simulink model "SMO_HFI_FOC"  (R2025b)
settings: Solver=FixedStepDiscrete  StartTime=0.0  StopTime=0.5  FixedStep=2e-05  RelTol=1e-3
settings Model: Creator=14420  LastModifiedBy=14420
settings DataIOCC: SaveOutput=off  SaveTime=off
settings DebuggingCC: AlgebraicLoopMsg=error

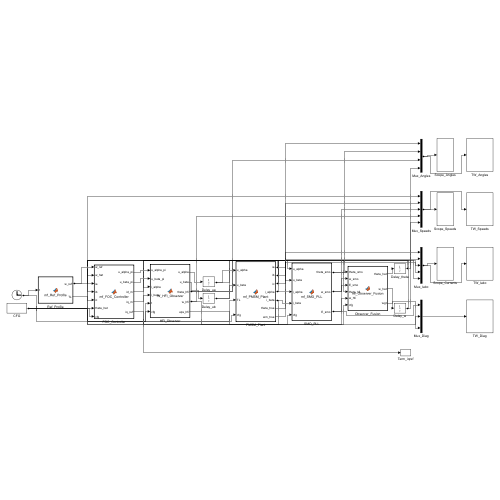
[thumbnail: Simulink's stored preview of the top-level diagram]
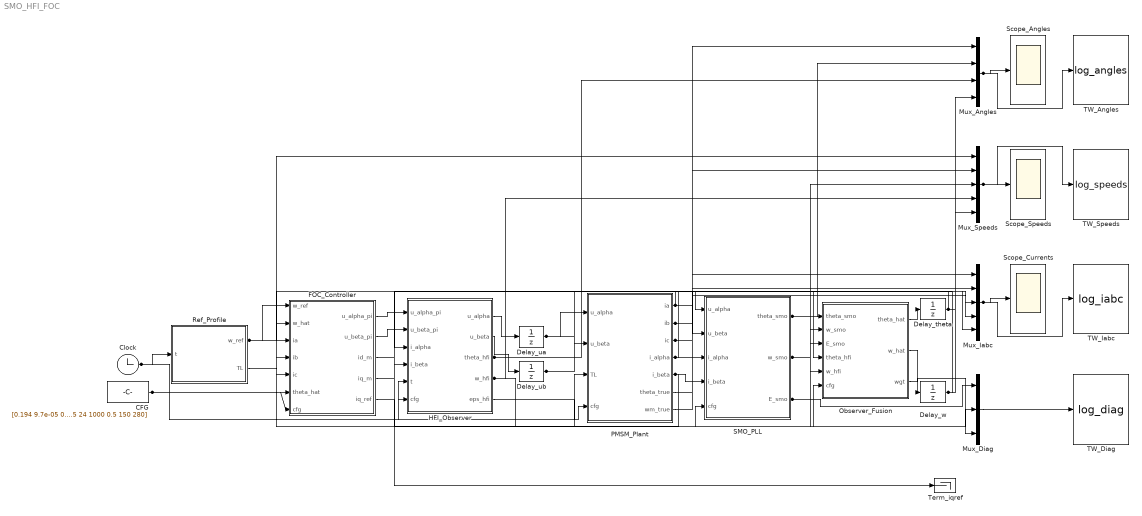
== system SMO_HFI_FOC ==
  CFG : Constant  Value=[0.194 9.7e-05 0.000145 0.015152 4 0.0006214 0.0003034 2e-05 24 1000 0.5 150 280]
  Clock : Clock
  Delay_theta : UnitDelay  SampleTime=2e-05  HasFrameUpgradeWarning=on
  Delay_ua : UnitDelay  SampleTime=2e-05  HasFrameUpgradeWarning=on
  Delay_ub : UnitDelay  SampleTime=2e-05  HasFrameUpgradeWarning=on
  Delay_w : UnitDelay  SampleTime=2e-05  HasFrameUpgradeWarning=on
  FOC_Controller : MATLAB Function  TreatAsAtomicUnit=on
  HFI_Observer : MATLAB Function  TreatAsAtomicUnit=on
  Mux_Angles : Mux
  Mux_Diag : Mux  Inputs=3
  Mux_Iabc : Mux  Inputs=5
  Mux_Speeds : Mux  Inputs=5
  Observer_Fusion : MATLAB Function  TreatAsAtomicUnit=on
  PMSM_Plant : MATLAB Function  TreatAsAtomicUnit=on
  Ref_Profile : MATLAB Function  TreatAsAtomicUnit=on
  SMO_PLL : MATLAB Function  TreatAsAtomicUnit=on
  Scope_Angles : Scope
  Scope_Currents : Scope
  Scope_Speeds : Scope
  TW_Angles : ToWorkspace  VariableName=log_angles  SaveFormat=Structure With Time  SampleTime=-1
  TW_Diag : ToWorkspace  VariableName=log_diag  SaveFormat=Structure With Time  SampleTime=-1
  TW_Iabc : ToWorkspace  VariableName=log_iabc  SaveFormat=Structure With Time  SampleTime=-1
  TW_Speeds : ToWorkspace  VariableName=log_speeds  SaveFormat=Structure With Time  SampleTime=-1
  Term_iqref : Terminator
  wires:
  Clock/1 -> Ref_Profile/1(t), HFI_Observer/5(t)
  CFG/1 -> FOC_Controller/7(cfg), HFI_Observer/6(cfg), PMSM_Plant/4(cfg), SMO_PLL/5(cfg), Observer_Fusion/6(cfg)
  Ref_Profile/1(w_ref) -> FOC_Controller/1(w_ref), Mux_Speeds/1
  Ref_Profile/2(TL) -> PMSM_Plant/3(TL)
  Observer_Fusion/1(theta_hat) -> Delay_theta/1
  Observer_Fusion/2(w_hat) -> Delay_w/1
  Delay_theta/1 -> FOC_Controller/6(theta_hat), Mux_Angles/4
  Delay_w/1 -> FOC_Controller/2(w_hat), Mux_Speeds/5
  Observer_Fusion/3(wgt) -> Mux_Diag/3
  FOC_Controller/1(u_alpha_pi) -> HFI_Observer/1(u_alpha_pi)
  FOC_Controller/2(u_beta_pi) -> HFI_Observer/2(u_beta_pi)
  FOC_Controller/5(iq_ref) -> Term_iqref/1
  FOC_Controller/3(id_m) -> Mux_Iabc/4
  FOC_Controller/4(iq_m) -> Mux_Iabc/5
  HFI_Observer/1(u_alpha) -> Delay_ua/1
  HFI_Observer/2(u_beta) -> Delay_ub/1
  HFI_Observer/3(theta_hfi) -> Mux_Angles/3, Observer_Fusion/4(theta_hfi)
  HFI_Observer/4(w_hfi) -> Observer_Fusion/5(w_hfi), Mux_Speeds/4
  HFI_Observer/5(eps_hfi) -> Mux_Diag/2
  Delay_ua/1 -> PMSM_Plant/1(u_alpha), SMO_PLL/1(u_alpha)
  Delay_ub/1 -> PMSM_Plant/2(u_beta), SMO_PLL/2(u_beta)
  PMSM_Plant/1(ia) -> FOC_Controller/3(ia), Mux_Iabc/1
  PMSM_Plant/2(ib) -> FOC_Controller/4(ib), Mux_Iabc/2
  PMSM_Plant/3(ic) -> FOC_Controller/5(ic), Mux_Iabc/3
  PMSM_Plant/4(i_alpha) -> SMO_PLL/3(i_alpha), HFI_Observer/3(i_alpha)
  PMSM_Plant/5(i_beta) -> SMO_PLL/4(i_beta), HFI_Observer/4(i_beta)
  PMSM_Plant/6(theta_true) -> Mux_Angles/1
  PMSM_Plant/7(wm_true) -> Mux_Speeds/2
  SMO_PLL/1(theta_smo) -> Mux_Angles/2, Observer_Fusion/1(theta_smo)
  SMO_PLL/2(w_smo) -> Observer_Fusion/2(w_smo), Mux_Speeds/3
  SMO_PLL/3(E_smo) -> Observer_Fusion/3(E_smo), Mux_Diag/1
  Mux_Angles/1 -> Scope_Angles/1, TW_Angles/1
  Mux_Speeds/1 -> Scope_Speeds/1, TW_Speeds/1
  Mux_Iabc/1 -> Scope_Currents/1, TW_Iabc/1
  Mux_Diag/1 -> TW_Diag/1

== matlab function SMO_HFI_FOC/FOC_Controller ==
  data: w_ref input; u_alpha_pi output; w_hat input; ia input; ib input; ic input; theta_hat input; cfg input; u_beta_pi output; id_m output; iq_m output; iq_ref output
function [u_alpha_pi, u_beta_pi, id_m, iq_m, iq_ref] = mf_FOC_Controller(w_ref, w_hat, ia, ib, ic, theta_hat, cfg)
%#codegen
% Speed loop (mechanical rad/s) plus the two current loops, all in the
% estimated dq frame.  cfg = [R Ld Lq psi pp J F Ts Udc fh Vh wlo whi].
R   = cfg(1);
Ld  = cfg(2);
Lq  = cfg(3);
psi = cfg(4);
pp  = cfg(5);
Ts  = cfg(8);
Udc = cfg(9);

% The speed loop must stay well below the observer bandwidth, otherwise it
% chases the injection PLL transients.
Kp_w  = 0.5;
Ki_w  = 5;
Kp_i  = 0.24;
Ki_i  = 490;
I_MAX = 4.0;

persistent xi_w int_d int_q
if isempty(xi_w)
    xi_w  = 0;
    int_d = 0;
    int_q = 0;
end

% ---- speed loop ----
e_w  = w_ref - w_hat;
xi_w = xi_w + Ki_w * e_w * Ts;
iq_c = Kp_w * e_w + xi_w;
if iq_c > I_MAX
    iq_c = I_MAX;
    xi_w = xi_w - Ki_w * e_w * Ts;
elseif iq_c < -I_MAX
    iq_c = -I_MAX;
    xi_w = xi_w - Ki_w * e_w * Ts;
end
iq_ref = iq_c;

% ---- Clarke, same convention as the plant ----
i_al = ia;
i_be = (ia + 2 * ib) / sqrt(3);

% ---- Park with the estimated angle ----
c = cos(theta_hat);
s = sin(theta_hat);
id_m =  i_al * c + i_be * s;
iq_m = -i_al * s + i_be * c;

% ---- current loops ----
e_d = 0 - id_m;
e_q = iq_ref - iq_m;
int_d = int_d + Ki_i * e_d * Ts;
int_q = int_q + Ki_i * e_q * Ts;
ud = Kp_i * e_d + int_d;
uq = Kp_i * e_q + int_q;

% ---- decoupling feed forward ----
we = pp * w_hat;
ud = ud - we * Lq * iq_m;
uq = uq + we * (Ld * id_m + psi);

% ---- linear modulation limit with back calculation ----
u_max = Udc / sqrt(3);
u_m   = sqrt(ud * ud + uq * uq);
if u_m > u_max
    k  = u_max / u_m;
    ud = ud * k;
    uq = uq * k;
    int_d = (ud + we * Lq * iq_m) - Kp_i * e_d;
    int_q = (uq - we * (Ld * id_m + psi)) - Kp_i * e_q;
end

% ---- inverse Park ----
u_alpha_pi = ud * c - uq * s;
u_beta_pi  = ud * s + uq * c;
end

== matlab function SMO_HFI_FOC/Ref_Profile ==
  data: t input; w_ref output; TL output
function [w_ref, TL] = mf_Ref_Profile(t)
%#codegen
% Mechanical speed reference [rad/s] and load torque [N m].
% 0.00 - 0.05 s : standstill, HFI has to hold the angle on its own
% 0.05 - 0.35 s : ramp up to 120 rad/s
% 0.35 - 0.50 s : hold, with a load torque step at 0.42 s
T_STAND = 0.05;
T_RAMP  = 0.35;
W_MAX   = 90;
T_LOAD  = 0.42;
TL_STEP = 0.03;

if t < T_STAND
    w_ref = 0;
elseif t < T_RAMP
    w_ref = W_MAX * (t - T_STAND) / (T_RAMP - T_STAND);
else
    w_ref = W_MAX;
end

if t >= T_LOAD
    TL = TL_STEP;
else
    TL = 0;
end
end

== matlab function SMO_HFI_FOC/HFI_Observer ==
  data: u_alpha_pi input; u_alpha output; u_beta_pi input; i_alpha input; i_beta input; t input; cfg input; u_beta output; theta_hfi output; w_hfi output; eps_hfi output
function [u_alpha, u_beta, theta_hfi, w_hfi, eps_hfi] = mf_HFI_Observer(u_alpha_pi, u_beta_pi, i_alpha, i_beta, t, cfg)
%#codegen
% Pulsating carrier injection along the estimated d axis, band pass around
% the carrier and synchronous demodulation of the q axis carrier current.
%   i_qh = Vh*(1/Ld-1/Lq)/(2*wh) * sin(2*dtheta) * sin(wh*t)
% The average of i_qh*sin(wh*t) over one carrier period gives
%   eps = Kth * sin(2*dtheta),  Kth = Vh*(1/Ld-1/Lq)/(4*wh)
% Two cascaded band pass sections centred exactly on the carrier remove the
% fundamental current, which is what otherwise swamps the demodulation as
% soon as the rotor turns.  A band pass has zero phase at its centre, so the
% demodulation stays in quadrature and the loop gain keeps its sign.
% N must equal 1/(fh*Ts).
Ld = cfg(2);
Lq = cfg(3);
Ts = cfg(8);
fh = cfg(10);
Vh = cfg(11);

WH     = 2 * pi * fh;
N      = 50;      % = 1/(fh*Ts)
QBP    = 3;       % band pass quality factor
W_GATE = 500;     % carrier is switched off above this electrical speed
KP_H   = 250;
KI_H   = 25000;
XI_MAX = 200;     % integrator limit: |w| stays below W_GATE so that the
                  % loop always keeps updating and can recover from a slip

persistent th w xi buf idx b0 b1 b2 a1 a2 x1 x2 y1 y2 x1b x2b y1b y2b
if isempty(th)
    th  = 0;
    w   = 0;
    xi  = 0;
    buf = zeros(N, 1);
    idx = 0;
    w0  = 2 * pi * fh * Ts;
    al  = sin(w0) / (2 * QBP);
    a0  = 1 + al;
    b0  = al / a0;
    b1  = 0;
    b2  = -al / a0;
    a1  = -2 * cos(w0) / a0;
    a2  = (1 - al) / a0;
    x1 = 0; x2 = 0; y1 = 0; y2 = 0;
    x1b = 0; x2b = 0; y1b = 0; y2b = 0;
end

if abs(w) > W_GATE
    Vh_e = 0;
else
    Vh_e = Vh;
end

c = cos(th);
s = sin(th);

% ---- carrier voltage along the estimated d axis ----
uc = Vh_e * cos(WH * t);
u_alpha = u_alpha_pi + uc * c;
u_beta  = u_beta_pi  + uc * s;

% ---- measured current in the estimated frame ----
id_h =  i_alpha * c + i_beta * s;
iq_h = -i_alpha * s + i_beta * c;

% ---- two cascaded band pass sections at the carrier ----
ys = b0 * iq_h + b1 * x1 + b2 * x2 - a1 * y1 - a2 * y2;
x2 = x1; x1 = iq_h; y2 = y1; y1 = ys;
yf = b0 * ys + b1 * x1b + b2 * x2b - a1 * y1b - a2 * y2b;
x2b = x1b; x1b = ys; y2b = y1b; y1b = yf;

% ---- synchronous demodulation, average over one carrier period ----
idx = idx + 1;
if idx > N
    idx = 1;
end
buf(idx) = yf * sin(WH * t);

acc = 0;
for k = 1:N
    acc = acc + buf(k);
end
eps_hfi = acc / N;

if abs(w) <= W_GATE
    Kth = Vh * (1 / Ld - 1 / Lq) / (4 * WH);
    if Kth == 0
        eps_n = 0;
    else
        eps_n = eps_hfi / Kth;
    end
    if eps_n >  1
        eps_n =  1;
    end
    if eps_n < -1
        eps_n = -1;
    end
    xi = xi + KI_H * eps_n * Ts;
    if xi >  XI_MAX
        xi =  XI_MAX;
    end
    if xi < -XI_MAX
        xi = -XI_MAX;
    end
    w  = KP_H * eps_n + xi;
    th = mod(th + w * Ts, 2 * pi);
end

theta_hfi = th;
w_hfi = w;
end

== matlab function SMO_HFI_FOC/PMSM_Plant ==
  data: u_alpha input; ia output; u_beta input; TL input; cfg input; ib output; ic output; i_alpha output; i_beta output; theta_true output; wm_true output
function [ia, ib, ic, i_alpha, i_beta, theta_true, wm_true] = mf_PMSM_Plant(u_alpha, u_beta, TL, cfg)
%#codegen
% Discrete dq model of a salient PMSM fed by an average value inverter.
% Forward Euler at Ts, currents and angle are states of the chart.
R  = cfg(1);
Ld = cfg(2);
Lq = cfg(3);
psi= cfg(4);
pp = cfg(5);
J  = cfg(6);
Ff = cfg(7);
Ts = cfg(8);

persistent id iq wm thm
if isempty(id)
    id = 0; iq = 0; wm = 0; thm = 0;
end

th_e = pp * thm;
c = cos(th_e);
s = sin(th_e);
ud =  u_alpha * c + u_beta * s;
uq = -u_alpha * s + u_beta * c;

we = pp * wm;
did = (ud - R * id + we * Lq * iq) / Ld;
diq = (uq - R * iq - we * Ld * id - we * psi) / Lq;
Te  = 1.5 * pp * (psi * iq + (Ld - Lq) * id * iq);
dwm = (Te - TL - Ff * wm) / J;

id  = id  + Ts * did;
iq  = iq  + Ts * diq;
wm  = wm  + Ts * dwm;
thm = thm + Ts * wm;

th_e = pp * thm;
c = cos(th_e);
s = sin(th_e);
i_alpha = id * c - iq * s;
i_beta  = id * s + iq * c;
ia = i_alpha;
ib = (sqrt(3) * i_beta - i_alpha) / 2;
ic = -ia - ib;

theta_true = mod(th_e, 2 * pi);
wm_true    = wm;
end

== matlab function SMO_HFI_FOC/SMO_PLL ==
  data: u_alpha input; theta_smo output; u_beta input; i_alpha input; i_beta input; cfg input; w_smo output; E_smo output
function [theta_smo, w_smo, E_smo] = mf_SMO_PLL(u_alpha, u_beta, i_alpha, i_beta, cfg)
%#codegen
% Sliding mode current observer in alpha beta plus a PLL on the estimated
% back EMF.  The PLL output is advanced by the phase lag of the back EMF
% low pass filter, otherwise the estimate would trail by atan(we/wc).
R  = cfg(1);
Ld = cfg(2);
Lq = cfg(3);
Ts = cfg(8);

L       = 0.5 * (Ld + Lq);
K_SLIDE = 40;
FC_EMF  = 200;
E_MIN   = 1.5;   % do not trust the EMF estimate while the carrier dominates
KP_PLL  = 300;
KI_PLL  = 20000;
XI_MAX  = 4000;

FC_W = 100;      % output speed filter [Hz]

persistent ia_h ib_h ea_f eb_f xi th w wf
if isempty(ia_h)
    ia_h = 0; ib_h = 0; ea_f = 0; eb_f = 0; xi = 0; th = 0; w = 0; wf = 0;
end

ea_r = ia_h - i_alpha;
eb_r = ib_h - i_beta;
za = K_SLIDE * sign(ea_r);
zb = K_SLIDE * sign(eb_r);

ia_h = ia_h + Ts * (u_alpha - R * ia_h - za) / L;
ib_h = ib_h + Ts * (u_beta  - R * ib_h - zb) / L;

al   = 1 - exp(-2 * pi * FC_EMF * Ts);
ea_f = (1 - al) * ea_f + al * za;
eb_f = (1 - al) * eb_f + al * zb;

E = sqrt(ea_f * ea_f + eb_f * eb_f);

if E > E_MIN
    eps_s = (-ea_f * cos(th) - eb_f * sin(th)) / E;
    xi = xi + KI_PLL * eps_s * Ts;
    if xi >  XI_MAX
        xi =  XI_MAX;
    end
    if xi < -XI_MAX
        xi = -XI_MAX;
    end
    w  = KP_PLL * eps_s + xi;
    th = th + w * Ts;
    th = mod(th, 2 * pi);
end

% The sliding mode term chatters, so the raw PLL speed is filtered before it
% leaves the observer.  The angle itself is an integral and stays smooth.
al_w = 2 * pi * FC_W * Ts;
wf   = wf + al_w * (w - wf);

theta_smo = mod(th + atan2(wf, 2 * pi * FC_EMF), 2 * pi);
w_smo = wf;
E_smo = E;
end

== matlab function SMO_HFI_FOC/Observer_Fusion ==
  data: theta_smo input; theta_hat output; w_smo input; E_smo input; theta_hfi input; w_hfi input; cfg input; w_hat output; wgt output
function [theta_hat, w_hat, wgt] = mf_Observer_Fusion(theta_smo, w_smo, E_smo, theta_hfi, w_hfi, cfg)
%#codegen
% Continuous fusion.  The injection observer owns standstill and low speed,
% the back EMF observer takes over as the flux linkage produces a usable EMF.
% The output angle is held by an NCO so that the output never jumps when the
% two inputs disagree, but the reported speed is the blended observer speed
% only: feeding the NCO trim back as speed would inject a phantom speed into
% the speed loop whenever the angle estimate is off.
psi  = cfg(4);
pp   = cfg(5);
Ts   = cfg(8);
% The membership is driven by the EMF magnitude, which grows monotonically
% with speed.  The old speed based test flickered because the SMO speed is
% noisy, and the flicker dragged the fused angle with it.
E1   = cfg(12) * psi;   % fade in  at this EMF [V]
E2   = cfg(13) * psi;   % fade out at this EMF [V]
E_OK = E1;
KNCO = 400;     % angle trimming gain [1/s]
WCMAX= 300;     % trim limit [electrical rad/s]
FC_W = 30;      % speed output filter [Hz]

persistent th wf
if isempty(th)
    th = theta_hfi;
    wf = 0;
end

if E_smo <= E1
    wgt = 0;
elseif E_smo >= E2
    wgt = 1;
else
    u   = (E_smo - E1) / (E2 - E1);
    wgt = u * u * (3 - 2 * u);
end

d_hfi = mod(theta_hfi - th + pi, 2 * pi) - pi;
d_smo = mod(theta_smo - th + pi, 2 * pi) - pi;

% The injection observer only resolves the rotor angle modulo pi.  As soon
% as the back EMF observer is trusted, the carrier estimate is aligned to the
% same pole: this is the standard way to remove the 180 deg ambiguity.
if (E_smo > E1) && (abs(d_hfi) > pi/2)
    d_hfi = mod(d_hfi + 2 * pi, 2 * pi) - pi;
end

w_obs  = (1 - wgt) * w_hfi + wgt * w_smo;
w_corr = KNCO * ((1 - wgt) * d_hfi + wgt * d_smo);
if w_corr >  WCMAX
    w_corr =  WCMAX;
end
if w_corr < -WCMAX
    w_corr = -WCMAX;
end

th = mod(th + (w_obs + w_corr) * Ts, 2 * pi);

% The reported speed is filtered: the injection loop has a fast, lightly
% damped speed channel and the speed regulator must not chase it.
al = 2 * pi * FC_W * Ts;
wf = wf + al * (w_obs - wf);

theta_hat = th;
w_hat     = wf / pp;
end
